simulink model "multiplier"  (R2021a)
settings: Solver=VariableStepAuto  StartTime=0.0  StopTime=10.0  RelTol=1e-3
libraries: custom_lib x18
settings Model: Creator=Acer  LastModifiedBy=Acer

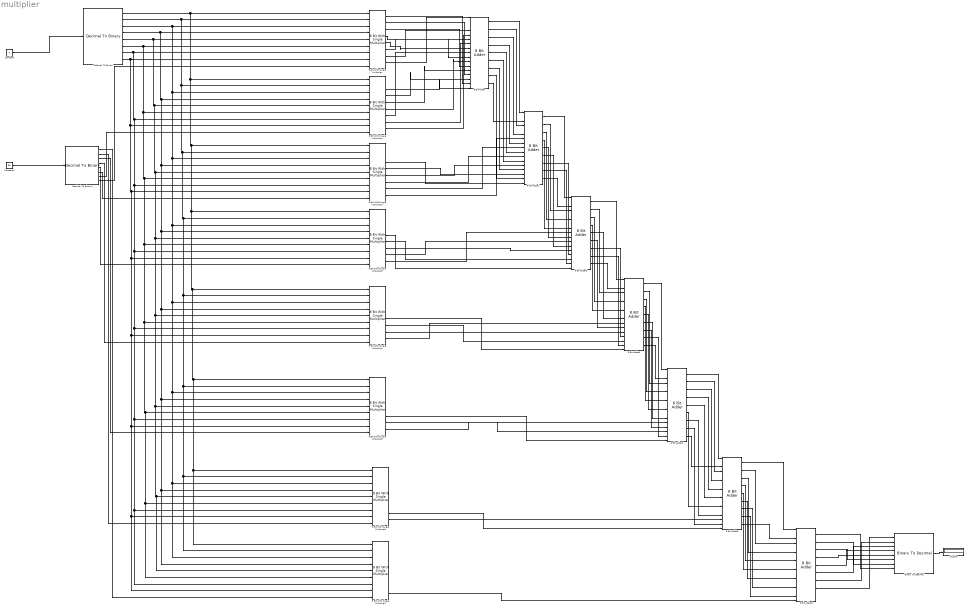
== system multiplier ==
  8 Bit Adder{,1..6} (7 alike) : custom_lib/8 Bit Adder  SystemSampleTime=-1  VariantActivationTime=update diagram  Latency=0  AutoFrameSizeCalculation=off
      settings: SourceProductName=Custom Library
  8 Bit With Single Multiplier{,1..7} (8 alike) : custom_lib/8 Bit With Single Multiplier  SystemSampleTime=-1  VariantActivationTime=update diagram  Latency=0  AutoFrameSizeCalculation=off
      settings: SourceProductName=Custom Library
  Binary To Decimal : custom_lib/Binary To Decimal  SystemSampleTime=-1  VariantActivationTime=update diagram  Latency=0  AutoFrameSizeCalculation=off
      settings: SourceProductName=Custom Library
  Constant : Constant  Value=0
  Constant1 : Constant  Value=99
  Decimal To Binary : custom_lib/Decimal To Binary  SystemSampleTime=-1  VariantActivationTime=update diagram  Latency=0  AutoFrameSizeCalculation=off
      settings: SourceProductName=Custom Library
  Decimal To Binary1 : custom_lib/Decimal To Binary  SystemSampleTime=-1  VariantActivationTime=update diagram  Latency=0  AutoFrameSizeCalculation=off
      settings: SourceProductName=Custom Library
  Display : Display
  wires:
  8 Bit With Single Multiplier/8 -> 8 Bit Adder/1
  8 Bit With Single Multiplier/7 -> 8 Bit Adder/4
  8 Bit With Single Multiplier/6 -> 8 Bit Adder/6
  8 Bit With Single Multiplier/5 -> 8 Bit Adder/8
  8 Bit With Single Multiplier/4 -> 8 Bit Adder/10
  8 Bit With Single Multiplier/3 -> 8 Bit Adder/12
  8 Bit With Single Multiplier/2 -> 8 Bit Adder/14
  8 Bit With Single Multiplier/1 -> 8 Bit Adder/16
  8 Bit With Single Multiplier1/8 -> 8 Bit Adder/5
  8 Bit With Single Multiplier1/7 -> 8 Bit Adder/7
  8 Bit With Single Multiplier1/6 -> 8 Bit Adder/9
  8 Bit With Single Multiplier1/5 -> 8 Bit Adder/11
  8 Bit With Single Multiplier1/4 -> 8 Bit Adder/13
  8 Bit With Single Multiplier1/3 -> 8 Bit Adder/15
  8 Bit With Single Multiplier1/2 -> 8 Bit Adder/17
  8 Bit Adder/9 -> 8 Bit Adder1/3
  8 Bit Adder/1 -> 8 Bit Adder1/1
  8 Bit Adder/2 -> 8 Bit Adder1/4
  8 Bit Adder/3 -> 8 Bit Adder1/6
  8 Bit Adder/4 -> 8 Bit Adder1/8
  8 Bit Adder/5 -> 8 Bit Adder1/10
  8 Bit Adder/6 -> 8 Bit Adder1/12
  8 Bit Adder/7 -> 8 Bit Adder1/14
  8 Bit Adder/8 -> 8 Bit Adder1/16
  8 Bit With Single Multiplier2/8 -> 8 Bit Adder1/7
  8 Bit With Single Multiplier2/7 -> 8 Bit Adder1/9
  8 Bit With Single Multiplier2/6 -> 8 Bit Adder1/11
  8 Bit With Single Multiplier2/5 -> 8 Bit Adder1/13
  8 Bit With Single Multiplier2/4 -> 8 Bit Adder1/15
  8 Bit With Single Multiplier2/3 -> 8 Bit Adder1/17
  8 Bit Adder1/9 -> 8 Bit Adder2/3
  8 Bit Adder1/1 -> 8 Bit Adder2/1
  8 Bit Adder1/2 -> 8 Bit Adder2/4
  8 Bit Adder1/3 -> 8 Bit Adder2/6
  8 Bit Adder1/4 -> 8 Bit Adder2/8
  8 Bit Adder1/5 -> 8 Bit Adder2/10
  8 Bit Adder1/6 -> 8 Bit Adder2/12
  8 Bit Adder1/7 -> 8 Bit Adder2/14
  8 Bit Adder1/8 -> 8 Bit Adder2/16
  8 Bit With Single Multiplier3/8 -> 8 Bit Adder2/9
  8 Bit With Single Multiplier3/7 -> 8 Bit Adder2/11
  8 Bit With Single Multiplier3/6 -> 8 Bit Adder2/13
  8 Bit With Single Multiplier3/5 -> 8 Bit Adder2/15
  8 Bit With Single Multiplier3/4 -> 8 Bit Adder2/17
  Constant/1 -> Decimal To Binary/1
  Constant1/1 -> Decimal To Binary1/1
  Decimal To Binary/8 -> 8 Bit With Single Multiplier7/8, 8 Bit With Single Multiplier6/8, 8 Bit With Single Multiplier5/8, 8 Bit With Single Multiplier4/8, 8 Bit With Single Multiplier3/8, 8 Bit With Single Multiplier2/8, 8 Bit With Single Multiplier1/8, 8 Bit With Single Multiplier/8
  Decimal To Binary/7 -> 8 Bit With Single Multiplier7/7, 8 Bit With Single Multiplier6/7, 8 Bit With Single Multiplier5/7, 8 Bit With Single Multiplier4/7, 8 Bit With Single Multiplier3/7, 8 Bit With Single Multiplier2/7, 8 Bit With Single Multiplier1/7, 8 Bit With Single Multiplier/7
  Decimal To Binary/6 -> 8 Bit With Single Multiplier7/6, 8 Bit With Single Multiplier6/6, 8 Bit With Single Multiplier5/6, 8 Bit With Single Multiplier4/6, 8 Bit With Single Multiplier3/6, 8 Bit With Single Multiplier2/6, 8 Bit With Single Multiplier1/6, 8 Bit With Single Multiplier/6
  Decimal To Binary/5 -> 8 Bit With Single Multiplier7/5, 8 Bit With Single Multiplier6/5, 8 Bit With Single Multiplier5/5, 8 Bit With Single Multiplier4/5, 8 Bit With Single Multiplier3/5, 8 Bit With Single Multiplier2/5, 8 Bit With Single Multiplier1/5, 8 Bit With Single Multiplier/5
  Decimal To Binary/4 -> 8 Bit With Single Multiplier7/4, 8 Bit With Single Multiplier6/4, 8 Bit With Single Multiplier5/4, 8 Bit With Single Multiplier4/4, 8 Bit With Single Multiplier3/4, 8 Bit With Single Multiplier2/4, 8 Bit With Single Multiplier1/4, 8 Bit With Single Multiplier/4
  Decimal To Binary/3 -> 8 Bit With Single Multiplier7/3, 8 Bit With Single Multiplier6/3, 8 Bit With Single Multiplier5/3, 8 Bit With Single Multiplier4/3, 8 Bit With Single Multiplier3/3, 8 Bit With Single Multiplier2/3, 8 Bit With Single Multiplier1/3, 8 Bit With Single Multiplier/3
  Decimal To Binary/2 -> 8 Bit With Single Multiplier7/2, 8 Bit With Single Multiplier6/2, 8 Bit With Single Multiplier5/2, 8 Bit With Single Multiplier4/2, 8 Bit With Single Multiplier3/2, 8 Bit With Single Multiplier2/2, 8 Bit With Single Multiplier1/2, 8 Bit With Single Multiplier/2
  Decimal To Binary/1 -> 8 Bit With Single Multiplier7/1, 8 Bit With Single Multiplier6/1, 8 Bit With Single Multiplier5/1, 8 Bit With Single Multiplier4/1, 8 Bit With Single Multiplier3/1, 8 Bit With Single Multiplier2/1, 8 Bit With Single Multiplier1/1, 8 Bit With Single Multiplier/1
  Decimal To Binary1/8 -> 8 Bit With Single Multiplier/9
  Decimal To Binary1/7 -> 8 Bit With Single Multiplier1/9
  Decimal To Binary1/6 -> 8 Bit With Single Multiplier2/9
  Decimal To Binary1/5 -> 8 Bit With Single Multiplier3/9
  8 Bit With Single Multiplier4/8 -> 8 Bit Adder3/11
  8 Bit With Single Multiplier4/7 -> 8 Bit Adder3/13
  8 Bit With Single Multiplier4/6 -> 8 Bit Adder3/15
  8 Bit With Single Multiplier4/5 -> 8 Bit Adder3/17
  8 Bit With Single Multiplier5/8 -> 8 Bit Adder4/13
  8 Bit With Single Multiplier5/7 -> 8 Bit Adder4/15
  8 Bit With Single Multiplier5/6 -> 8 Bit Adder4/17
  8 Bit With Single Multiplier6/8 -> 8 Bit Adder5/15
  8 Bit With Single Multiplier6/7 -> 8 Bit Adder5/17
  8 Bit With Single Multiplier7/8 -> 8 Bit Adder6/17
  8 Bit Adder2/9 -> 8 Bit Adder3/3
  8 Bit Adder2/1 -> 8 Bit Adder3/1
  8 Bit Adder2/2 -> 8 Bit Adder3/4
  8 Bit Adder2/3 -> 8 Bit Adder3/6
  8 Bit Adder2/4 -> 8 Bit Adder3/8
  8 Bit Adder2/5 -> 8 Bit Adder3/10
  8 Bit Adder2/6 -> 8 Bit Adder3/12
  8 Bit Adder2/7 -> 8 Bit Adder3/14
  8 Bit Adder2/8 -> 8 Bit Adder3/16
  8 Bit Adder3/9 -> 8 Bit Adder4/3
  8 Bit Adder3/1 -> 8 Bit Adder4/1
  8 Bit Adder3/2 -> 8 Bit Adder4/4
  8 Bit Adder3/3 -> 8 Bit Adder4/6
  8 Bit Adder3/4 -> 8 Bit Adder4/8
  8 Bit Adder3/5 -> 8 Bit Adder4/10
  8 Bit Adder3/6 -> 8 Bit Adder4/12
  8 Bit Adder3/7 -> 8 Bit Adder4/14
  8 Bit Adder3/8 -> 8 Bit Adder4/16
  8 Bit Adder4/9 -> 8 Bit Adder5/3
  8 Bit Adder4/1 -> 8 Bit Adder5/1
  8 Bit Adder4/2 -> 8 Bit Adder5/4
  8 Bit Adder4/3 -> 8 Bit Adder5/6
  8 Bit Adder4/4 -> 8 Bit Adder5/8
  8 Bit Adder4/5 -> 8 Bit Adder5/10
  8 Bit Adder4/6 -> 8 Bit Adder5/12
  8 Bit Adder4/7 -> 8 Bit Adder5/14
  8 Bit Adder4/8 -> 8 Bit Adder5/16
  8 Bit Adder5/9 -> 8 Bit Adder6/3
  8 Bit Adder5/1 -> 8 Bit Adder6/1
  8 Bit Adder5/2 -> 8 Bit Adder6/4
  8 Bit Adder5/3 -> 8 Bit Adder6/6
  8 Bit Adder5/4 -> 8 Bit Adder6/8
  8 Bit Adder5/5 -> 8 Bit Adder6/10
  8 Bit Adder5/6 -> 8 Bit Adder6/12
  8 Bit Adder5/7 -> 8 Bit Adder6/14
  8 Bit Adder5/8 -> 8 Bit Adder6/16
  8 Bit Adder6/1 -> Binary To Decimal/8
  8 Bit Adder6/2 -> Binary To Decimal/7
  8 Bit Adder6/3 -> Binary To Decimal/6
  8 Bit Adder6/4 -> Binary To Decimal/5
  8 Bit Adder6/5 -> Binary To Decimal/4
  8 Bit Adder6/6 -> Binary To Decimal/3
  8 Bit Adder6/7 -> Binary To Decimal/2
  8 Bit Adder6/8 -> Binary To Decimal/1
  Binary To Decimal/1 -> Display/1
  Decimal To Binary1/4 -> 8 Bit With Single Multiplier4/9
  Decimal To Binary1/3 -> 8 Bit With Single Multiplier5/9
  Decimal To Binary1/2 -> 8 Bit With Single Multiplier6/9
  Decimal To Binary1/1 -> 8 Bit With Single Multiplier7/9
